simulink model "regulate_tank"  (R2023a)
settings: Solver=VariableStepAuto  StartTime=0.0  StopTime=T  RelTol=1e-3
values from neighbouring files (symbols this model uses):
  A = 1    [regulate_tank_script.m]
  h_ref = 0.5    [regulate_tank_script.m]
  k = 1    [regulate_tank_script.m]
  Ki = 0.1    [regulate_tank_script.m]
  Kp = 100    [regulate_tank_script.m]
  rho = 1000    [regulate_tank_script.m]
  w = 0    [regulate_tank_script.m]
undefined symbols (not defined in the file or in its folder): tau
settings Model: Creator=eriknymobohne  LastModifiedBy=eriknymobohne

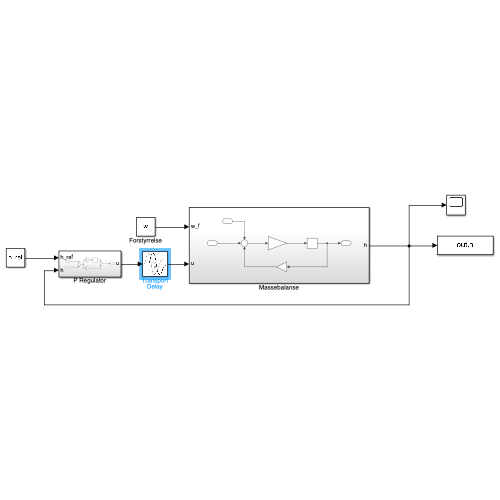
[thumbnail: Simulink's stored preview of the top-level diagram]
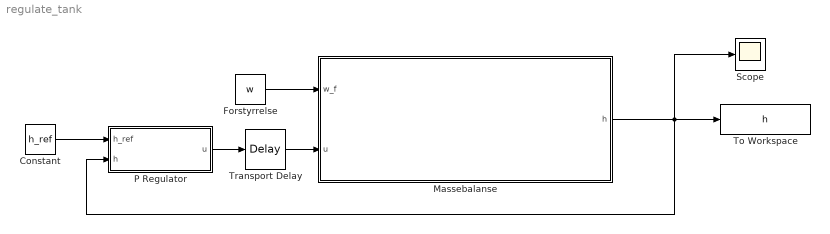
== system regulate_tank ==
  Constant : Constant  Value=h_ref
  Forstyrrelse : Constant  Value=w
  Massebalanse : Subsystem
  P Regulator : Subsystem
  Scope : Scope
  To Workspace : ToWorkspace  VariableName=h  SaveFormat=Timeseries  SampleTime=-1
  Transport Delay : TransportDelay  DelayTime=tau
  wires:
  Massebalanse/1(h) -> P Regulator/2(h), To Workspace/1, Scope/1
  Constant/1 -> P Regulator/1(h_ref)
  Forstyrrelse/1 -> Massebalanse/1(w_f)
  P Regulator/1(u) -> Transport Delay/1
  Transport Delay/1 -> Massebalanse/2(u)

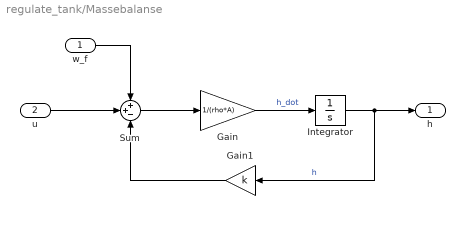
== system regulate_tank/Massebalanse ==
  w_f : Inport
  u : Inport  Port=2
  Gain : Gain  Gain=1/(rho*A)
  Gain1 : Gain  Gain=k
  Integrator : Integrator
  Sum : Sum  Inputs=++-
  h : Outport
  wires:
  u/1 -> Sum/2
  Integrator/1 -> h/1, Gain1/1  "h"
  Sum/1 -> Gain/1
  Gain1/1 -> Sum/3
  Gain/1 -> Integrator/1  "h_dot"
  w_f/1 -> Sum/1

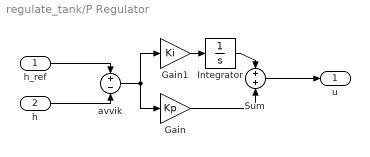
== system regulate_tank/P Regulator ==
  h_ref : Inport
  h : Inport  Port=2
  Gain : Gain  Gain=Kp
  Gain1 : Gain  Gain=Ki
  Integrator : Integrator
  Sum : Sum  Inputs=+|+
  avvik : Sum  Inputs=+|-
  u : Outport
  wires:
  h_ref/1 -> avvik/1
  h/1 -> avvik/2
  avvik/1 -> Gain1/1, Gain/1
  Sum/1 -> u/1
  Gain/1 -> Sum/2
  Gain1/1 -> Integrator/1
  Integrator/1 -> Sum/1
